simulink model "SIM"  (R2018b)
settings: Solver=VariableStepAuto  StartTime=0.0  StopTime=20  RelTol=1e-3  EnableMultiTasking=on
values from neighbouring files (symbols this model uses):
  A_lat = [-2*kD*Vbz/m  0                 0                -g*C_GAM(3,2)/m                             -g*C_PSI(3,2)/m  0;         0           0                 (Jyy-Jzz)*Wz/Jxx  0                                           0               0;         0           (Jzz-Jxx)*Wz/Jyy  0                 0 0 0;         0           1                -cos(GAM)*tan(TET) Wz*cos(GAM)*tan(TET)+Wy*sin(GAM)*tan(TET)   0     ...(+251 chars)    [LINEARIZATION_NEW.m]
  B_lat = [0 0; 1/Jxx 0; 0 1/Jyy; 0 0; 0 0; 0 0;]    [LINEARIZATION_NEW.m]
  C_long = [0 0 0 1 0 0]    [LINEARIZATION_NEW.m]
settings Model: Creator=XINGAU  LastModifiedBy=diepn
settings DataIOCC: LimitDataPoints=on
settings OptimizationCC: LifeSpan=inf
settings DebuggingCC: AllowSymbolicDim=off  SFUnexpectedBacktrackingDiag=warning  SFNoUnconditionalDefaultTransitionDiag=warning  SFExecutionAtInitializationDiag=none
settings ModelReferenceCC: PropagateSignalLabelsOutOfModel=off
settings SFSimCC: SimUseLocalCustomCode=off
settings RTWCC: RTWUseLocalCustomCode=off
settings CodeAppCC: StateflowObjectComments=on
settings GRTTargetCC: TargetLangStandard=C89/C90 (ANSI)
settings ConfigComp: CovMetricSettings=dw  CovHtmlReporting=on  CovSaveCumulativeToWorkspaceVar=on  CovSaveSingleToWorkspaceVar=on  CovExternalEMLEnable=off

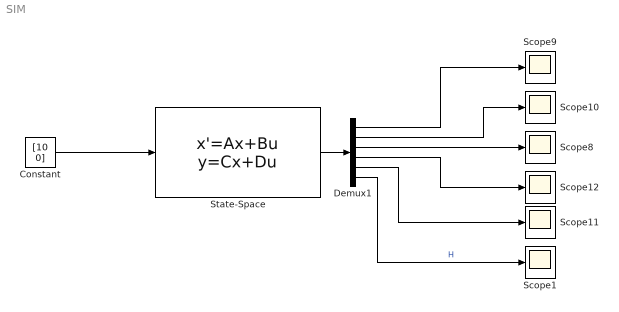
== system SIM ==
  Constant : Constant  Value=[10 0]
  Demux1 : Demux  Outputs=6
  Scope{1,8..12} (6 alike) : Scope
  State-Space : StateSpace  A=A_lat  B=B_lat  C=C_long  D=zeros(6,2)  InitialCondition=[0 0 0 0 0 0]'
  wires:
  State-Space/1 -> Demux1/1
  Demux1/3 -> Scope8/1
  Demux1/1 -> Scope9/1
  Demux1/2 -> Scope10/1
  Demux1/4 -> Scope12/1
  Demux1/5 -> Scope11/1
  Constant/1 -> State-Space/1
  Demux1/6 -> Scope1/1  "H"
